simulink model "main"  (R2023b)
settings: Solver=VariableStepAuto  StartTime=0.0  StopTime=10.0  RelTol=1e-3
settings Model: Creator=han  LastModifiedBy=han

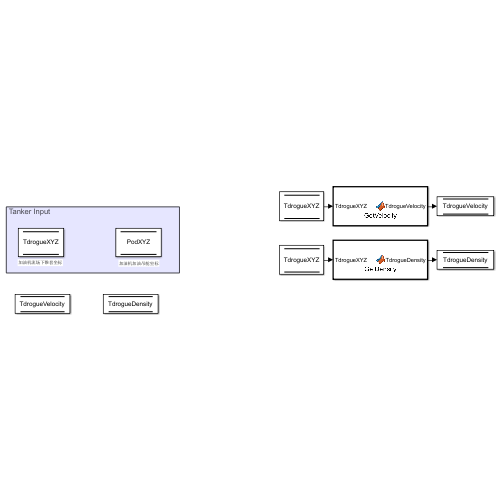
[thumbnail: Simulink's stored preview of the top-level diagram]
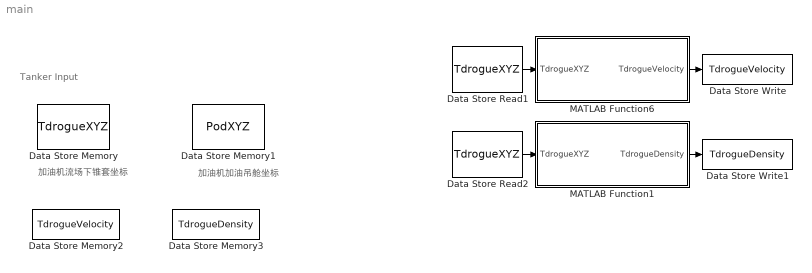
== system main ==
  note: Tanker Input
  note: 加油机加油吊舱坐标
  note: 加油机流场下锥套坐标
  Data Store Memory : DataStoreMemory  DataStoreName=TdrogueXYZ  WriteAfterWriteMsg=warning  InitialValue=TdrogueXYZ0  ShowAdditionalParam=off
  Data Store Memory1 : DataStoreMemory  DataStoreName=PodXYZ  WriteAfterWriteMsg=warning  InitialValue=PodXYZ  ShowAdditionalParam=off
  Data Store Memory2 : DataStoreMemory  DataStoreName=TdrogueVelocity  WriteAfterWriteMsg=warning  InitialValue=[0,0,0]  ShowAdditionalParam=off
  Data Store Memory3 : DataStoreMemory  DataStoreName=TdrogueDensity  WriteAfterWriteMsg=warning  ShowAdditionalParam=off
  Data Store Read1 : DataStoreRead  DataStoreName=TdrogueXYZ  IndexOptions=Index vector (dialog)  Indices=1  OutputSizes=1
  Data Store Read2 : DataStoreRead  DataStoreName=TdrogueXYZ  IndexOptions=Index vector (dialog)  Indices=1  OutputSizes=1
  Data Store Write : DataStoreWrite  DataStoreName=TdrogueVelocity  IndexOptions=Index vector (dialog)  Indices=1  OutputSizes=1
  Data Store Write1 : DataStoreWrite  DataStoreName=TdrogueDensity  IndexOptions=Index vector (dialog)  Indices=1  OutputSizes=1
  MATLAB Function1 : MATLAB Function  TreatAsAtomicUnit=on
  MATLAB Function6 : MATLAB Function  TreatAsAtomicUnit=on
  wires:
  Data Store Read1/1 -> MATLAB Function6/1(TdrogueXYZ)
  MATLAB Function6/1(TdrogueVelocity) -> Data Store Write/1
  Data Store Read2/1 -> MATLAB Function1/1(TdrogueXYZ)
  MATLAB Function1/1(TdrogueDensity) -> Data Store Write1/1

== matlab function main/MATLAB Function6 ==
  data: TdrogueVelocity output; TdrogueXYZ input
function TdrogueVelocity = GetVelocity(TdrogueXYZ)
coder.extrinsic("py.pyvista")
coder.extrinsic("py.numpy")
coder.extrinsic("py.ReadData.py")
coder.extrinsic("py.ReadData.get_velocity")
TdrogueVelocity = [0.0,0.0,0.0];
TdrogueVelocity = double(py.ReadData.get_velocity(TdrogueXYZ(1),TdrogueXYZ(2),TdrogueXYZ(3)));

== matlab function main/MATLAB Function1 ==
  data: TdrogueDensity output; TdrogueXYZ input
function TdrogueDensity = GetDensity(TdrogueXYZ)
coder.extrinsic("py.pyvista")
coder.extrinsic("py.numpy")
coder.extrinsic("py.ReadData.py")
coder.extrinsic("py.ReadData.get_density")
TdrogueDensity = 0.0;
TdrogueDensity = double(py.ReadData.get_density(TdrogueXYZ(1),TdrogueXYZ(2),TdrogueXYZ(3)));
